simulink model "step1_geo_sband_link_system"  (R2026a)
settings: Solver=FixedStepDiscrete  StopTime=1  FixedStep=1
settings Model: Creator=24470  LastModifiedBy=24470

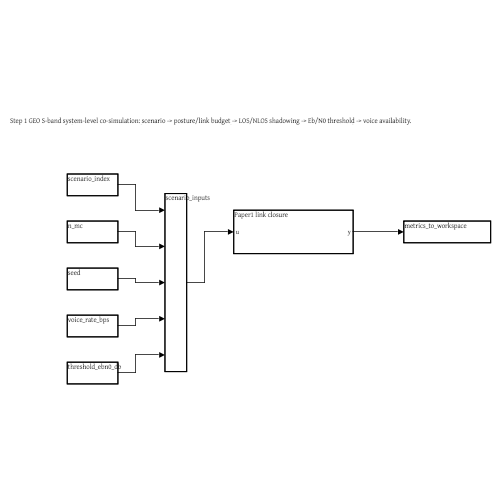
[thumbnail: Simulink's stored preview of the top-level diagram]
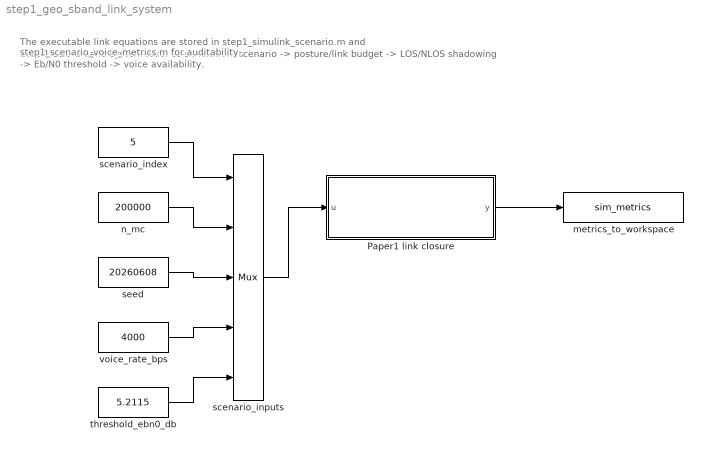
== system step1_geo_sband_link_system ==
  note: Step 1 GEO S-band system-level co-simulation: scenario -> posture/link budget -> LOS/NLOS shadowing -> Eb/N0 threshold -> voice availability.
  note: The executable link equations are stored in step1_simulink_scenario.m and step1_scenario_voice_metrics.m for auditability.
  Paper1 link closure : MATLAB Function  TreatAsAtomicUnit=on
  metrics_to_workspace : ToWorkspace  VariableName=sim_metrics  SampleTime=-1
  n_mc : Constant  Value=200000
  scenario_index : Constant  Value=5
  scenario_inputs : Mux  Inputs=5
  seed : Constant  Value=20260608
  threshold_ebn0_db : Constant  Value=5.2115
  voice_rate_bps : Constant  Value=4000
  wires:
  scenario_index/1 -> scenario_inputs/1
  n_mc/1 -> scenario_inputs/2
  seed/1 -> scenario_inputs/3
  voice_rate_bps/1 -> scenario_inputs/4
  threshold_ebn0_db/1 -> scenario_inputs/5
  scenario_inputs/1 -> Paper1 link closure/1(u)
  Paper1 link closure/1(y) -> metrics_to_workspace/1

== matlab function step1_geo_sband_link_system/Paper1 link closure ==
  data: u input; y output
function y = fcn(u)
%#codegen
coder.extrinsic('step1_simulink_scenario');
y = zeros(9,1);
y = step1_simulink_scenario(u);
end
